simulink model "model1"  (Simulink 7.3)
settings: Solver=ode45  StartTime=0.0  StopTime=5  RelTol=1e-3
settings Model: Creator=IEUser  LastModifiedBy=IEUser

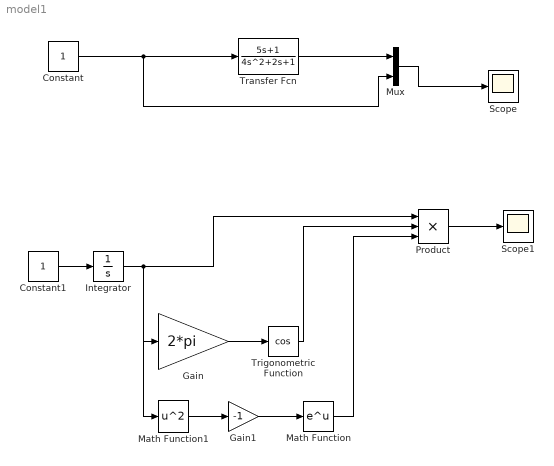
== system model1 ==
  Constant : Constant  OutDataType=fixdt(1, 16)  OutScaling=2^0
  Constant1 : Constant  OutDataType=fixdt(1, 16)  OutScaling=2^0
  Gain : Gain  Gain=2*pi  ParameterDataType=fixdt(1, 16)  ParameterScaling=2^0  OutDataType=fixdt(1, 16)  OutScaling=2^0
  Gain1 : Gain  Gain=-1  ParameterDataType=fixdt(1, 16)  ParameterScaling=2^0  OutDataType=fixdt(1, 16)  OutScaling=2^0
  Integrator : Integrator
  Math Function : Math  OutDataType=fixdt(1, 16)  OutScaling=2^0  SaturateOnIntegerOverflow=on
  Math Function1 : Math  Operator=square  OutDataType=fixdt(1, 16)  OutScaling=2^0  SaturateOnIntegerOverflow=on
  Mux : Mux  Inputs=2
  Product : Product  Inputs=3  OutDataType=fixdt(1, 16)  OutScaling=2^0  RndMeth=Zero
  Scope : Scope
  Scope1 : Scope
  Transfer Fcn : TransferFcn  Numerator=[5 1]  Denominator=[4 2 1]
  Trigonometric Function : Trigonometry  Operator=cos
  wires:
  Constant/1 -> Transfer Fcn/1, Mux/2
  Transfer Fcn/1 -> Mux/1
  Mux/1 -> Scope/1
  Constant1/1 -> Integrator/1
  Integrator/1 -> Gain/1, Math Function1/1, Product/1
  Gain/1 -> Trigonometric Function/1
  Trigonometric Function/1 -> Product/2
  Product/1 -> Scope1/1
  Math Function/1 -> Product/3
  Math Function1/1 -> Gain1/1
  Gain1/1 -> Math Function/1
